simulink model "model2"  (R2024b)
settings: Solver=VariableStepAuto  StartTime=0.0  StopTime=10.0  RelTol=1e-3
undefined symbols (not defined in the file): c, k, m
settings Model: Creator=kacpe  LastModifiedBy=kacpe

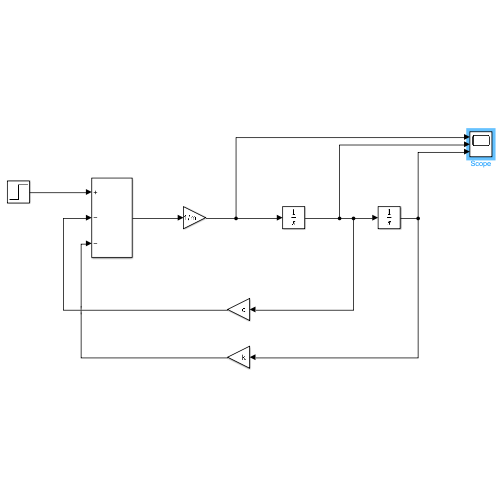
[thumbnail: Simulink's stored preview of the top-level diagram]
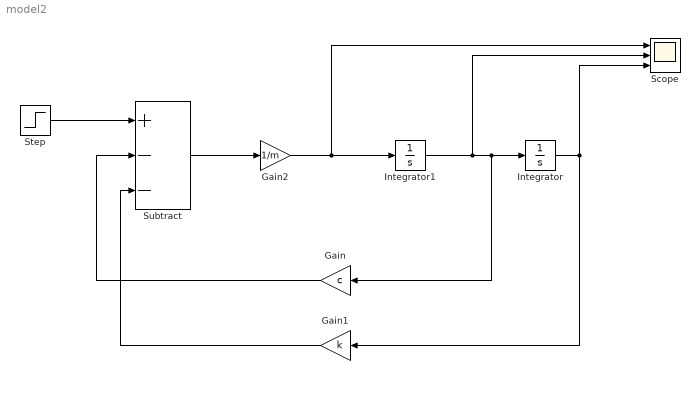
== system model2 ==
  Gain : Gain  Gain=c
  Gain1 : Gain  Gain=k
  Gain2 : Gain  Gain=1/m
  Integrator : Integrator
  Integrator1 : Integrator
  Scope : Scope  NumInputPorts=3
  Step : Step  After=25  SampleTime=0
  Subtract : Sum  Inputs=+--
  wires:
  Step/1 -> Subtract/1
  Subtract/1 -> Gain2/1
  Gain2/1 -> Scope/1, Integrator1/1
  Integrator1/1 -> Scope/2, Gain/1, Integrator/1
  Integrator/1 -> Gain1/1, Scope/3
  Gain1/1 -> Subtract/3
  Gain/1 -> Subtract/2
